simulink model "QCar2_DetailedScenario-2025a"  (R2025a)
settings: Solver=ode2  StartTime=0.0  StopTime=inf  FixedStep=1/100  RelTol=1e-3  EnableMultiTasking=on
model workspace (MAT data in the model file):
  XY_OFFSET : Simulink.Parameter (value not decoded)
  camera_rate : Simulink.Parameter (value not decoded)
  depth_rate : Simulink.Parameter (value not decoded)
  path_to_pickup : Simulink.Parameter (value not decoded)
  path_to_pickup_tight : Simulink.Parameter (value not decoded)
symbols that are objects in the model workspace (value not decoded): camera_rate, depth_rate, path_to_pickup, XY_OFFSET
undefined symbols (not defined in the file or in its folder): gcbh, HIL, JPEG, Point, qc_get_step_size, Video3D, video_display_show
libraries: quarc_library x37, simulink x16
(part 2 of 3)

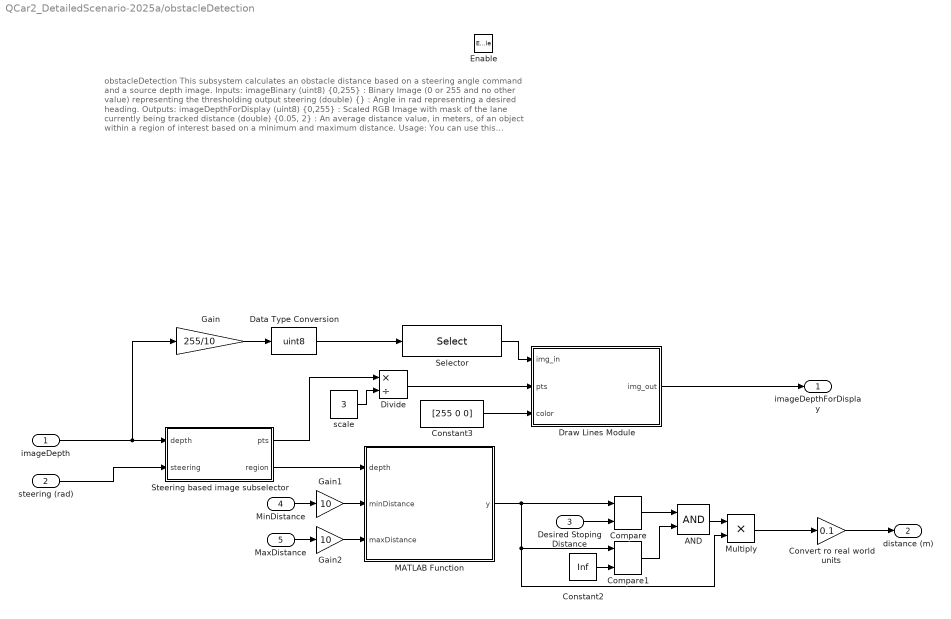
== system QCar2_DetailedScenario-2025a/obstacleDetection ==
  note: obstacleDetection
      | This subsystem calculates an obstacle distance based on a steering angle command and a source depth image.
      |
      | Inputs:
      | imageBinary (uint8) {0,255} : Binary Image (0 or 255 and no other value) representing the thresholding output
      | steering (double) {} : Angle in rad representing a desired heading.
      |
      | Outputs:
      | imageDepthForDisplay (uint8) {0,255} : Scaled RGB Image with mask of the lane currently being tracked
      | distance (double) {0.05, 2} : An average distance value, in meters, of an object within a region of interest based on a minimum and maximum distance.
      |
      | Usage:
      |
      | You can use this subsystem to determine if the desired heading angle will cause the car to colllide with an obstacle by examining the distances from a region of interest within the depth image and calculating how far the obstacle is.
  imageDepth : Inport
  steering (rad) : Inport  Port=2
  Desired Stoping Distance : Inport  Port=3
  MinDistance : Inport  Port=4
  MaxDistance : Inport  Port=5
  Enable : EnablePort  PropagateVarSize=During execution
  AND : Logic  AllPortsSameDT=off  OutDataTypeStr=boolean
  Compare : quarc_library/Logic Operations/Compare  operator=>=  output_data_type=boolean
      settings: SourceProductName=QUARC Targets
  Compare1 : quarc_library/Logic Operations/Compare  operator=<  output_data_type=boolean
      settings: SourceProductName=QUARC Targets
  Constant2 : Constant  Value=Inf
  Constant3 : Constant  Value=[255 0 0]
  Convert ro real world units : Gain  Gain=0.1
  Data Type Conversion : DataTypeConversion  OutDataTypeStr=uint8  SaturateOnIntegerOverflow=off  RndMeth=Floor
  Divide : Product  Inputs=*/  OutDataTypeStr=Inherit: Inherit via back propagation
  Draw Lines Module : MATLAB Function  TreatAsAtomicUnit=on
  Gain : Gain  Gain=255/10
  Gain1 : Gain  Gain=10
  Gain2 : Gain  Gain=10
  MATLAB Function : MATLAB Function  TreatAsAtomicUnit=on
  Multiply : Product
  Selector : Selector  NumberOfDimensions=2  InputPortWidth=3  IndexOptions=Index vector (dialog),Index vector (dialog)  Indices=[1:3:360],[1:3:640]  OutputSizes=1,1
  Steering based image subselector : MATLAB Function  TreatAsAtomicUnit=on
  scale : Constant  Value=3
  imageDepthForDisplay : Outport  VectorParamsAs1DForOutWhenUnconnected=off
  distance (m) : Outport  Port=2  VectorParamsAs1DForOutWhenUnconnected=off
  wires:
  Constant3/1 -> Draw Lines Module/3(color)
  Steering based image subselector/1(pts) -> Divide/1
  Steering based image subselector/2(region) -> MATLAB Function/1(depth)
  steering (rad)/1 -> Steering based image subselector/2(steering)
  Multiply/1 -> Convert ro real world units/1
  MaxDistance/1 -> Gain2/1
  MinDistance/1 -> Gain1/1
  MATLAB Function/1(y) -> Compare/1, Multiply/2, Compare1/1
  imageDepth/1 -> Steering based image subselector/1(depth), Gain/1
  Selector/1 -> Draw Lines Module/1(img_in)
  Data Type Conversion/1 -> Selector/1
  Divide/1 -> Draw Lines Module/2(pts)
  Draw Lines Module/1(img_out) -> imageDepthForDisplay/1
  scale/1 -> Divide/2
  Gain/1 -> Data Type Conversion/1
  Desired Stoping Distance/1 -> Compare/2
  Compare/1 -> AND/1
  Compare1/1 -> AND/2
  Constant2/1 -> Compare1/2
  AND/1 -> Multiply/1
  Convert ro real world units/1 -> distance (m)/1
  Gain1/1 -> MATLAB Function/2(minDistance)
  Gain2/1 -> MATLAB Function/3(maxDistance)

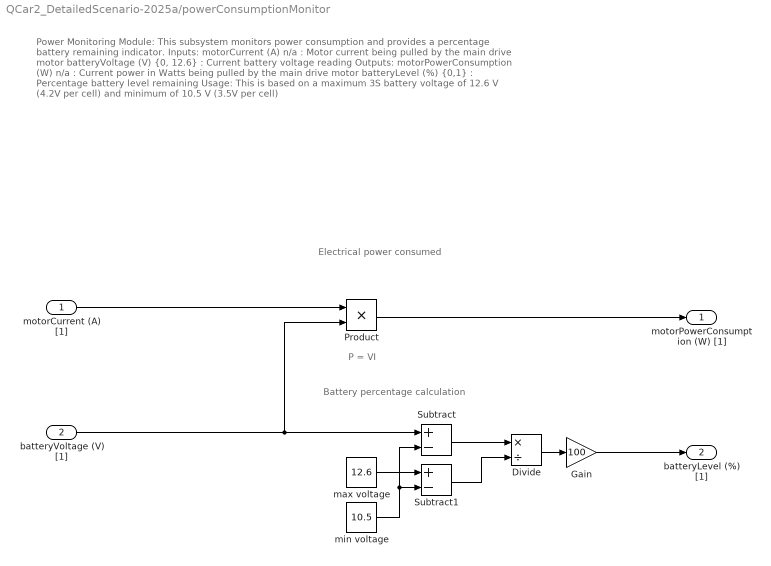
== system QCar2_DetailedScenario-2025a/powerConsumptionMonitor ==
  note: Battery percentage calculation
  note: P = VI
  note: Electrical
      | power
      | consumed
  note: Power Monitoring Module:
      |
      | This subsystem monitors power consumption and provides a percentage battery remaining indicator.
      |
      | Inputs:
      | motorCurrent (A) n/a : Motor current being pulled by the main drive motor
      | batteryVoltage (V) {0, 12.6} : Current battery voltage reading
      |
      | Outputs:
      | motorPowerConsumption (W) n/a : Current power in Watts being pulled by the main drive motor
      | batteryLevel (%) {0,1} : Percentage battery level remaining
      |
      | Usage:
      | This is based on a maximum 3S battery voltage of 12.6 V (4.2V per cell) and minimum of 10.5 V (3.5V per cell)
  motorCurrent (A) [1] : Inport
  batteryVoltage (V) [1] : Inport  Port=2
  Divide : Product  Inputs=*/
  Gain : Gain  Gain=100
  Product : Product
  Subtract : Sum  Inputs=+-
  Subtract1 : Sum  Inputs=+-
  max voltage : Constant  Value=12.6
  min voltage : Constant  Value=10.5
  motorPowerConsumption (W) [1] : Outport  VectorParamsAs1DForOutWhenUnconnected=off
  batteryLevel (%) [1] : Outport  Port=2  VectorParamsAs1DForOutWhenUnconnected=off
  wires:
  Divide/1 -> Gain/1
  Subtract1/1 -> Divide/2
  Gain/1 -> batteryLevel (%) [1]/1
  Product/1 -> motorPowerConsumption (W) [1]/1
  min voltage/1 -> Subtract/2, Subtract1/2
  motorCurrent (A) [1]/1 -> Product/1
  max voltage/1 -> Subtract1/1
  Subtract/1 -> Divide/1
  batteryVoltage (V) [1]/1 -> Subtract/1, Product/2

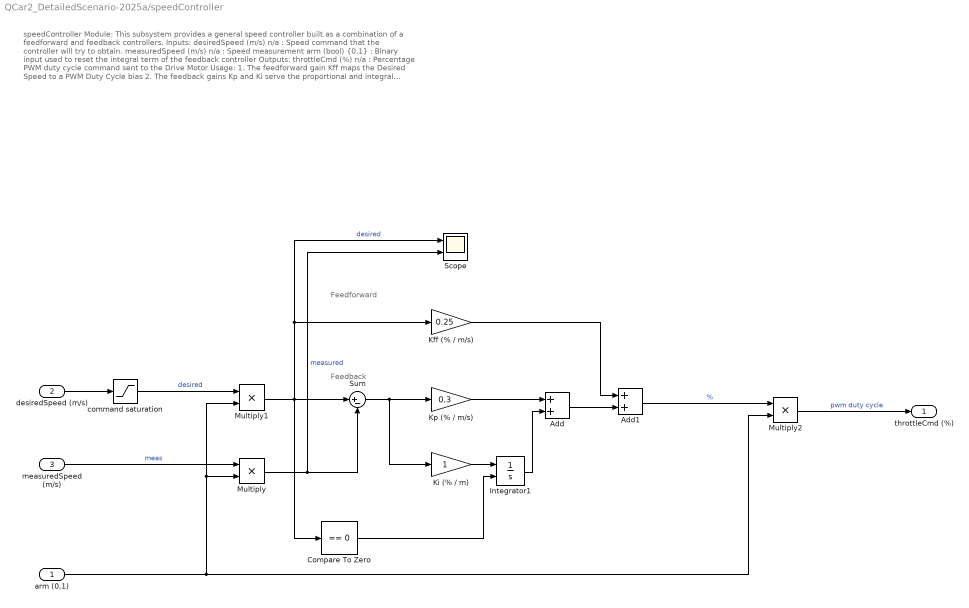
== system QCar2_DetailedScenario-2025a/speedController ==
  note: Feedforward
  note: Feedback
  note: speedController Module:
      |
      | This subsystem provides a general speed controller built as a combination of a feedforward and feedback controllers.
      |
      | Inputs:
      | desiredSpeed (m/s) n/a : Speed command that the controller will try to obtain.
      | measuredSpeed (m/s) n/a : Speed measurement
      | arm (bool) {0,1} : Binary input used to reset the integral term of the feedback controller
      |
      | Outputs:
      | throttleCmd (%) n/a : Percentage PWM duty cycle command sent to the Drive Motor
      |
      | Usage:
      | 1. The feedforward gain Kff maps the Desired Speed to a PWM Duty Cycle bias
      | 2. The feedback gains Kp and Ki serve the proportional and integral terms to output corrections to the PWM Duty Cycle so as to regulate the desired speed.
  arm (0,1) : Inport
  desiredSpeed (m/s) : Inport  Port=2
  measuredSpeed (m/s) : Inport  Port=3
  Add : Sum
  Add1 : Sum
  Compare To Zero : simulink/Logic and Bit Operations/Compare To Zero  relop===  OutDataTypeStr=boolean
  Integrator1 : Integrator  ExternalReset=either  LimitOutput=on  UpperSaturationLimit=0.4  LowerSaturationLimit=-0.4
  Kff (% / m/s) : Gain  Gain=0.25
  "Ki (% / m) " : Gain
  Kp (% / m/s) : Gain  Gain=0.3
  Multiply : Product
  Multiply1 : Product
  Multiply2 : Product
  Scope : Scope  NumInputPorts=2
      settings: Title=Control Performance  ActiveDisplayYMinimum=1.4224  ActiveDisplayYMaximum=2.10565  YLabel=m/s
  Sum : Sum  Inputs=|+-
  command saturation : Saturate  UpperLimit=5  LowerLimit=-5
  throttleCmd (%) : Outport  VectorParamsAs1DForOutWhenUnconnected=off
  wires:
  command saturation/1 -> Multiply1/1  "desired"
  arm (0,1)/1 -> Multiply1/2, Multiply/2, Multiply2/2
  measuredSpeed (m/s)/1 -> Multiply/1  "meas"
  Multiply/1 -> Sum/2, Scope/2  "measured"
  Add/1 -> Add1/2
  Add1/1 -> Multiply2/1  "%"
  Multiply1/1 -> Compare To Zero/1, Sum/1, Kff (% / m/s)/1, Scope/1  "desired"
  Integrator1/1 -> Add/2
  Multiply2/1 -> throttleCmd (%)/1  "pwm duty cycle"
  Kp (% / m/s)/1 -> Add/1
  Compare To Zero/1 -> Integrator1/2
  Kff (% / m/s)/1 -> Add1/1
  Sum/1 -> "Ki (% / m) "/1, Kp (% / m/s)/1
  "Ki (% / m) "/1 -> Integrator1/1
  desiredSpeed (m/s)/1 -> command saturation/1

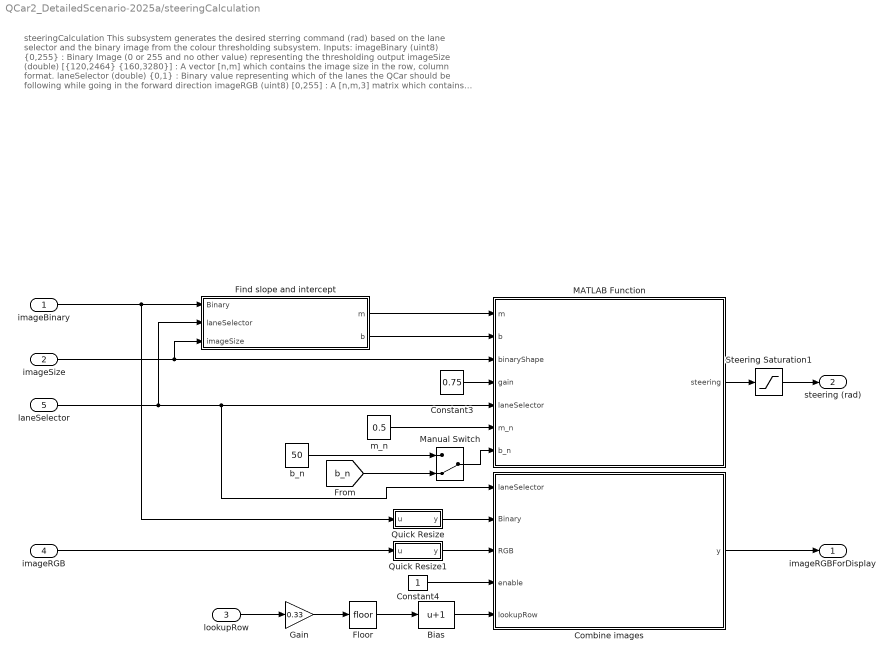
== system QCar2_DetailedScenario-2025a/steeringCalculation ==
  note: steeringCalculation
      | This subsystem generates the desired sterring command (rad) based on the lane selector and the binary image from the colour thresholding subsystem.
      |
      | Inputs:
      | imageBinary (uint8) {0,255} : Binary Image (0 or 255 and no other value) representing the thresholding output
      | imageSize (double) [{120,2464} {160,3280}] : A vector [n,m] which contains the image size in the row, column format.
      | laneSelector (double) {0,1} : Binary value representing which of the lanes the QCar should be following while going in the forward direction
      | imageRGB (uint8) [0,255] : A [n,m,3] matrix which contains RGB values of an image in uint8 format
      |
      | Outputs:
      | steering (double) {-0.5,0.5} : Angle in rad representing the desired steering command based on the linearPolyFit
      | imageRGBForDisplay (uint8) {0,255} : A [n,m,3] matrix representing an RGB Image with mask of the lane currently being tracked
      |
      | Usage:
      |
      | This module can be used to generate a desired steering angle based on a thresheld image. A linear polygonal fit is used to generate a slope based on the equation y = mx+b whose slope and y intercept will define the steering angle commanded up to 0.5 (rad). The RGB image is a combination of the binary image holding information of the lane being followed, and a scaled version of the original RGB image.
  imageBinary : Inport
  imageSize : Inport  Port=2
  lookupRow : Inport  Port=3
  imageRGB : Inport  Port=4
  laneSelector : Inport  Port=5
  Bias : Bias  Bias=1  SaturateOnIntegerOverflow=off
  Combine images : MATLAB Function  TreatAsAtomicUnit=on
  Constant3 : Constant  Value=0.75
  Constant4 : Constant
  Find slope and intercept : MATLAB Function  TreatAsAtomicUnit=on
  Floor : Rounding
  Gain : Gain  Gain=0.33
  MATLAB Function : MATLAB Function  TreatAsAtomicUnit=on
  Manual Switch : ManualSwitch  CurrentSetting=0
  Quick Resize : MATLAB Function  TreatAsAtomicUnit=on
  Quick Resize1 : MATLAB Function  TreatAsAtomicUnit=on
  Steering Saturation1 : Saturate
  b_n : Constant  Value=50
  m_n : Constant  Value=0.5
  imageRGBForDisplay : Outport  VectorParamsAs1DForOutWhenUnconnected=off
  steering (rad) : Outport  Port=2  VectorParamsAs1DForOutWhenUnconnected=off
  wires:
  Find slope and intercept/1(m) -> MATLAB Function/1(m)
  laneSelector/1 -> MATLAB Function/5(laneSelector), Combine images/1(laneSelector), Find slope and intercept/2(laneSelector)
  MATLAB Function/1(steering) -> Steering Saturation1/1
  Constant3/1 -> MATLAB Function/4(gain)
  imageBinary/1 -> Quick Resize/1(u), Find slope and intercept/1(Binary)
  Find slope and intercept/2(b) -> MATLAB Function/2(b)
  Constant4/1 -> Combine images/4(enable)
  Quick Resize/1(y) -> Combine images/2(Binary)
  Quick Resize1/1(y) -> Combine images/3(RGB)
  Combine images/1(y) -> imageRGBForDisplay/1
  imageRGB/1 -> Quick Resize1/1(u)
  Steering Saturation1/1 -> steering (rad)/1
  Gain/1 -> Floor/1
  imageSize/1 -> Find slope and intercept/3(imageSize), MATLAB Function/3(binaryShape)
  lookupRow/1 -> Gain/1
  Bias/1 -> Combine images/5(lookupRow)
  Floor/1 -> Bias/1
  b_n/1 -> Manual Switch/1
  Manual Switch/1 -> MATLAB Function/7(b_n)
  [b_n] -> Manual Switch/2
  m_n/1 -> MATLAB Function/6(m_n)

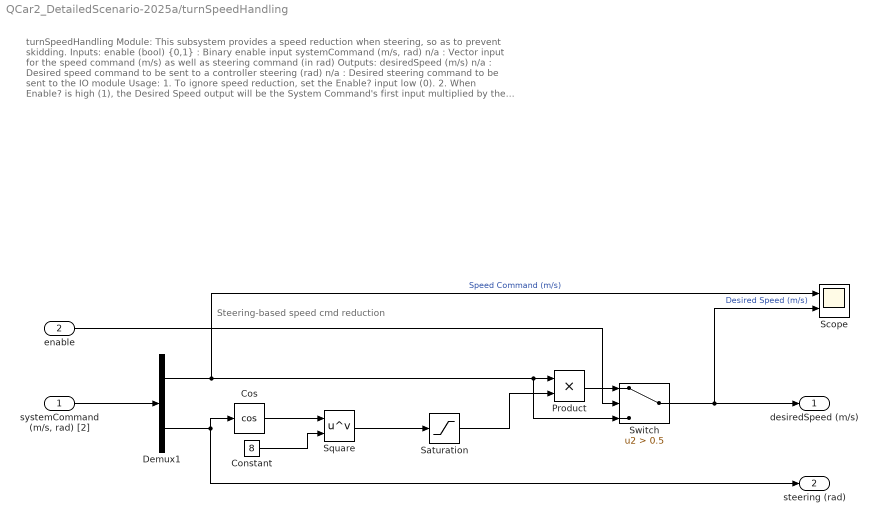
== system QCar2_DetailedScenario-2025a/turnSpeedHandling ==
  note: turnSpeedHandling Module:
      |
      | This subsystem provides a speed reduction when steering, so as to prevent skidding.
      |
      | Inputs:
      | enable (bool) {0,1} : Binary enable input
      | systemCommand (m/s, rad) n/a : Vector input for the speed command (m/s) as well as steering command (in rad)
      |
      | Outputs:
      | desiredSpeed (m/s) n/a : Desired speed command to be sent to a controller
      | steering (rad) n/a : Desired steering command to be sent to the IO module
      |
      | Usage:
      | 1. To ignore speed reduction, set the Enable? input low (0).
      | 2. When Enable? is high (1), the Desired Speed output will be the System Command's first input multiplied by the cosine of the steering. Note that the lower limit of this reduction is set to 50% of the speed command input.
  note: Steering-based speed cmd reduction
  "systemCommand (m/s, rad) [2]" : Inport
  enable : Inport  Port=2
  Constant : Constant  Value=8
  Cos : Trigonometry  Operator=cos
  Demux1 : Demux  Outputs=2
  Product : Product
  Saturation : Saturate  UpperLimit=1  LowerLimit=0.5
  Scope : Scope  NumInputPorts=2
      settings: Title=Turn-Speed Handling  ActiveDisplayYMinimum=-2  ActiveDisplayYMaximum=2  YLabel=m/s  DataLoggingVariableName=ScopeData2
  Square : Math  Operator=pow  SignedPower=on
  Switch : Switch  Criteria=u2 > Threshold  Threshold=0.5  SaturateOnIntegerOverflow=off  InputSameDT=off
  desiredSpeed (m/s) : Outport  VectorParamsAs1DForOutWhenUnconnected=off
  steering (rad) : Outport  Port=2  VectorParamsAs1DForOutWhenUnconnected=off
  wires:
  Cos/1 -> Square/1
  Switch/1 -> desiredSpeed (m/s)/1, Scope/2  "Desired Speed (m/s)"
  Product/1 -> Switch/1
  Saturation/1 -> Product/2
  Demux1/1 -> Product/1, Switch/3, Scope/1  "Speed Command (m/s)"
  "systemCommand (m/s, rad) [2]"/1 -> Demux1/1
  enable/1 -> Switch/2
  Constant/1 -> Square/2
  Demux1/2 -> steering (rad)/1, Cos/1
  Square/1 -> Saturation/1

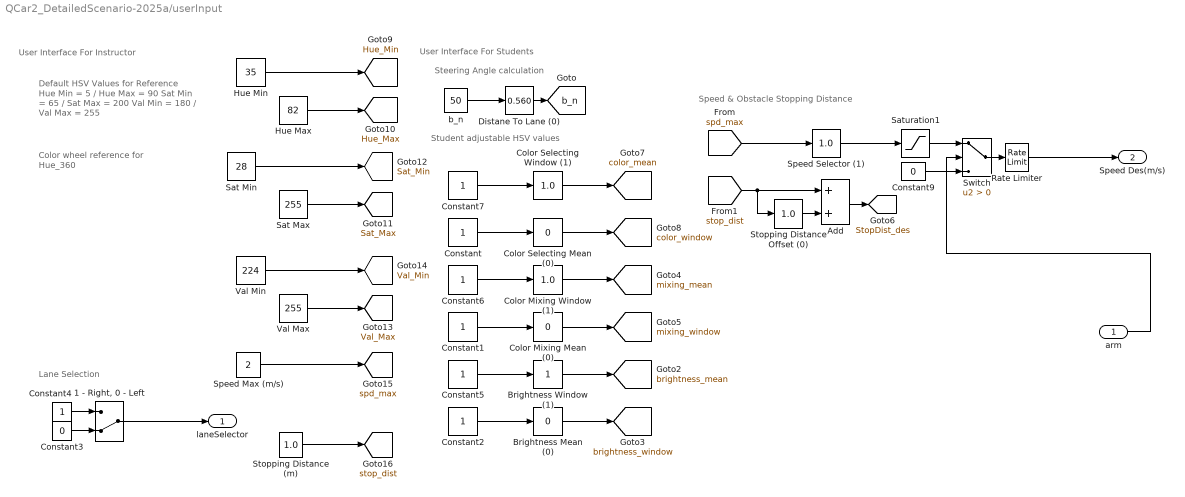
== system QCar2_DetailedScenario-2025a/userInput ==
  note: Default HSV Values for Reference
      | Hue Min = 5 / Hue Max = 90
      | Sat Min = 65 / Sat Max = 200
      | Val Min = 180 / Val Max = 255
  note: User Interface For Instructor
  note: Student adjustable HSV values
  note: Lane Selection
  note: Steering Angle calculation
  note: User Interface For Students
  note: Speed & Obstacle Stopping Distance
  note: Color wheel
      | reference
      | for Hue_360
  arm : Inport  OutDataTypeStr=boolean
  "1 - Right, 0 - Left" : ManualSwitch  CurrentSetting=0
  Add : Sum
  Brightness Mean (0) : simulink/Math Operations/Slider Gain  gain=0  low=-1  high=1
  Brightness Window (1) : simulink/Math Operations/Slider Gain  gain=1  low=0  high=1
  Color Mixing Mean (0) : simulink/Math Operations/Slider Gain  gain=0  low=-1  high=1
  Color Mixing Window (1) : simulink/Math Operations/Slider Gain  gain=1.0  low=0  high=1
  Color Selecting Mean (0) : simulink/Math Operations/Slider Gain  gain=0  low=-1  high=1
  Color Selecting Window (1) : simulink/Math Operations/Slider Gain  gain=1.0  low=0  high=1
  Constant{,1..2,4..7} (7 alike) : Constant
  Constant3 : Constant  Value=0
  Constant9 : Constant  Value=0
  "Distane To Lane (0) " : simulink/Math Operations/Slider Gain  gain=0.560  low=0  high=1
  Hue Max : Constant  Value=82
  Hue Min : Constant  Value=35
  Rate Limiter : RateLimiter  FallingSlewLimit=-Inf  SampleTimeMode=inherited
  Sat Max : Constant  Value=255
  Sat Min : Constant  Value=28
  Saturation1 : Saturate  UpperLimit=1  LowerLimit=0
  Speed Max (m/s) : Constant  Value=2
  Speed Selector (1) : simulink/Math Operations/Slider Gain  gain=1.0  low=0  high=1
  Stopping Distance (m) : Constant  Value=1.0
  Stopping Distance Offset (0) : simulink/Math Operations/Slider Gain  gain=1.0  low=0  high=1
  Switch : Switch  Criteria=u2 > Threshold  SaturateOnIntegerOverflow=off  InputSameDT=off
  Val Max : Constant  Value=255
  Val Min : Constant  Value=224
  b_n : Constant  Value=50
  laneSelector : Outport  VectorParamsAs1DForOutWhenUnconnected=off
  Speed Des(m/s) : Outport  Port=2  VectorParamsAs1DForOutWhenUnconnected=off
  tag scope: Hue_Max=global, Hue_Min=global, Sat_Max=global, Sat_Min=global, StopDist_des=global, Val_Max=global, Val_Min=global, b_n=global, brightness_mean=global, brightness_window=global, color_mean=global, color_window=global, mixing_mean=global, mixing_window=global, spd_max=global, stop_dist=global
  wires:
  Constant3/1 -> "1 - Right, 0 - Left"/2
  b_n/1 -> "Distane To Lane (0) "/1
  Constant4/1 -> "1 - Right, 0 - Left"/1
  Switch/1 -> Rate Limiter/1
  Constant9/1 -> Switch/3
  [spd_max] -> Speed Selector (1)/1
  Saturation1/1 -> Switch/1
  "1 - Right, 0 - Left"/1 -> laneSelector/1
  Rate Limiter/1 -> Speed Des(m/s)/1
  "Distane To Lane (0) "/1 -> [b_n]
  Color Mixing Window (1)/1 -> [mixing_mean]
  Constant/1 -> Color Selecting Mean (0)/1
  Constant2/1 -> Brightness Mean (0)/1
  Constant5/1 -> Brightness Window (1)/1
  Constant1/1 -> Color Mixing Mean (0)/1
  Color Selecting Mean (0)/1 -> [color_window]
  Brightness Window (1)/1 -> [brightness_mean]
  Color Selecting Window (1)/1 -> [color_mean]
  Brightness Mean (0)/1 -> [brightness_window]
  Color Mixing Mean (0)/1 -> [mixing_window]
  Constant6/1 -> Color Mixing Window (1)/1
  Constant7/1 -> Color Selecting Window (1)/1
  Hue Min/1 -> [Hue_Min]
  Sat Min/1 -> [Sat_Min]
  Val Min/1 -> [Val_Min]
  Hue Max/1 -> [Hue_Max]
  Sat Max/1 -> [Sat_Max]
  Val Max/1 -> [Val_Max]
  Speed Selector (1)/1 -> Saturation1/1
  Speed Max (m/s)/1 -> [spd_max]
  Stopping Distance (m)/1 -> [stop_dist]
  [stop_dist] -> Stopping Distance Offset (0)/1, Add/1
  Stopping Distance Offset (0)/1 -> Add/2
  Add/1 -> [StopDist_des]
  arm/1 -> Switch/2

== system QCar2_DetailedScenario-2025a/basicQCarIO/Video Compressed Display ==
  In1 : Inport
  Channel : quarc_library/Signal Routing/Channel  channel=3  buffer_size=1
  Image Compress : quarc_library/Image Processing/Generic/Image Compress  algorithm=JPEG  source=Internal dialog parameter  quality=quality  output_dim=-1
  Video Display : quarc_library/Multimedia/Video Display  Tag=QCar2_DetailedScenario/basicQCarIO/Video Compressed Display/Video Display  sample_time=sample_time  use_hardware=on
  wires:
  Image Compress/1 -> Channel/1
  In1/1 -> Image Compress/1
  Channel/1 -> Video Display/1

== system QCar2_DetailedScenario-2025a/basicQCarIO/captureLIDAR ==
  note: captureLIDAR Module:
      |
      | This subsystem reads the LIDAR data from the QCar. This module reads 720 points per revolution at 30 Hz (30 scans per s).
      |
      | Outputs:
      | distances (m) n/a : Distances to obstacles measured
      | headings (rad) n/a : Headings at which distances were measured
  note: LIDAR Capture, and heading adjustment
  "Change +x to front of QCar " : Bias  SaturateOnIntegerOverflow=off
  Change to CCW rotation : Gain  Gain=-1
  Ranging Sensor : quarc_library/Devices/Third-Party/Sensors/Ranging Sensor  sensor_type=RPLidar LIDAR  uri=tcpip://localhost:18966  ranging_distance=Long  timing_budget=0.033  measurement_period=0.0001  output_mode=Fixed-size output  samples_per_revolution=360  max_distance=Inf  max_angle=5  sample_time=qc_get_step_size  show_versions=off  active=on
      settings: SourceProductName=QUARC Targets
  Terminator{,1..3} (4 alike) : Terminator
  distances (m) : Outport  VectorParamsAs1DForOutWhenUnconnected=off
  headings (rad) : Outport  Port=2  VectorParamsAs1DForOutWhenUnconnected=off
  wires:
  Ranging Sensor/1 -> distances (m)/1
  "Change +x to front of QCar "/1 -> headings (rad)/1
  Ranging Sensor/3 -> Change to CCW rotation/1
  Ranging Sensor/2 -> Terminator/1
  Change to CCW rotation/1 -> "Change +x to front of QCar "/1
  Ranging Sensor/5 -> Terminator3/1
  Ranging Sensor/6 -> Terminator1/1
  Ranging Sensor/4 -> Terminator2/1

== system QCar2_DetailedScenario-2025a/basicQCarIO/monitorTiming  ==
  note: Timing Performance
  note: monitorTiming Module:
      |
      | This subsystem provides three timing signals for any given rate in your model.
      |
      | Outputs:
      | timing (s) n/a : Sample time, sample time reference and computation time in seconds.
      |
      | Usage:
      | Set the 'Sample time (seconds)' parameter in all three blocks below to the same number. This will provide the actual sample time at each time step, the reference sample time that is being targeted as well as the computation time of that particular loop in the model into one vector signal for scoping.
  Computation Time : quarc_library/Sources/Time/Computation Time  sample_time=qc_get_step_size  use_model=on  use_cpu_time=off
  Constant : Constant  Value=qc_get_step_size
  Mux : Mux  Inputs=3
  Sample Time : quarc_library/Sources/Time/Sample Time  Priority=-99  sample_time=qc_get_step_size
  timing (s) : Outport  VectorParamsAs1DForOutWhenUnconnected=off
  wires:
  Mux/1 -> timing (s)/1
  Computation Time/1 -> Mux/3  "computation time"
  Sample Time/1 -> Mux/1  "actual sample time"
  Constant/1 -> Mux/2  "reference"

== system QCar2_DetailedScenario-2025a/basicQCarIO/odometry ==
  v_in : Inport
  steer_in : Inport  Port=2
  Ts_const : Constant  Value=0.02
  odometry_step : MATLAB Function  TreatAsAtomicUnit=on
  state_delay : UnitDelay  InitialCondition=[0;0;0]  SampleTime=-1  HasFrameUpgradeWarning=on
  pose_out : Outport
  wires:
  state_delay/1 -> odometry_step/1(prev_state)
  v_in/1 -> odometry_step/2(v)
  steer_in/1 -> odometry_step/3(steer)
  Ts_const/1 -> odometry_step/4(Ts)
  odometry_step/1(pose_next) -> state_delay/1, pose_out/1

== system QCar2_DetailedScenario-2025a/basicQCarIO/pointCloud ==
  note: Convert LIDAR information to Point Cloud Image
  note: pointCloud Module:
      |
      | This subsystem generates a point cloud image based on LIDAR data.
      |
      | Inputs:
      | distances (m) n/a : Distances measured by LIDAR
      | headings (rad) n/a : Headings at which distances are measured
      |
      | Outputs:
      | map (px) {0, 1} : 400 x 400 point cloud image
      |
      | Usage:
      | The data is dynamically saturated based on the maximumDistance (m) constant. To prevent a circle with radius being the maximumDistance showing up in the point cloud as a result of this saturation, data points corresponding to this are dropped in the findXYContour function. The function contourToPointCloud updates pixels in the map to 1 at new locations, and decays older data at the rate specified by the decay parameter.
  distances (m) : Inport
  heading (rad) : Inport  Port=2
  Constant1 : Constant  Value=0
  Saturation Dynamic : simulink/Discontinuities/Saturation Dynamic  OutMin=[]  OutMax=[]  OutDataTypeStr=Inherit: Same as second input  OutDataType=fixdt(1, 16)  OutScaling=2^-10  DoSatur=off
  contourToPointCloud : MATLAB Function  TreatAsAtomicUnit=on
  decay : Constant  Value=0
  findXYContour : MATLAB Function  TreatAsAtomicUnit=on
  maximumDistance (m) : Constant  Value=4
  map : Outport  VectorParamsAs1DForOutWhenUnconnected=off
  wires:
  distances (m)/1 -> Saturation Dynamic/2
  contourToPointCloud/1(mapOut) -> map/1
  Saturation Dynamic/1 -> findXYContour/1(distances)
  maximumDistance (m)/1 -> findXYContour/3(d_max), Saturation Dynamic/1
  Constant1/1 -> Saturation Dynamic/3
  decay/1 -> contourToPointCloud/3(decay)
  findXYContour/1(X) -> contourToPointCloud/1(X)
  findXYContour/2(Y) -> contourToPointCloud/2(Y)
  heading (rad)/1 -> findXYContour/2(heading)

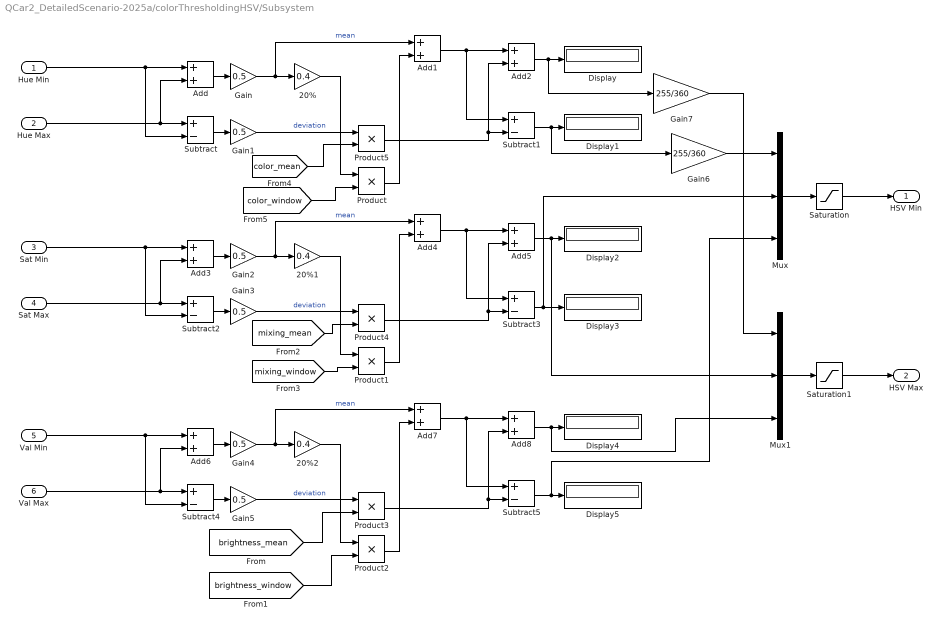
== system QCar2_DetailedScenario-2025a/colorThresholdingHSV/Subsystem ==
  Hue Min : Inport
  Hue Max : Inport  Port=2
  Sat Min : Inport  Port=3
  Sat Max : Inport  Port=4
  Val Min : Inport  Port=5
  Val Max : Inport  Port=6
  20% : Gain  Gain=0.4
  20%1 : Gain  Gain=0.4
  20%2 : Gain  Gain=0.4
  Add{,1..8} (9 alike) : Sum
  Display{,1..5} (6 alike) : Display
  Gain{,1..5} (6 alike) : Gain  Gain=0.5
  Gain6 : Gain  Gain=255/360
  Gain7 : Gain  Gain=255/360
  Mux : Mux  Inputs=3
  Mux1 : Mux  Inputs=3
  Product{,1..5} (6 alike) : Product
  Saturation : Saturate  UpperLimit=[255 255 255]  LowerLimit=[0 0 0]
  Saturation1 : Saturate  UpperLimit=[255 255 255]  LowerLimit=[0 0 0]
  Subtract{,1..5} (6 alike) : Sum  Inputs=+-
  HSV Min : Outport  VectorParamsAs1DForOutWhenUnconnected=off
  HSV Max : Outport  Port=2  VectorParamsAs1DForOutWhenUnconnected=off
  wires:
  Product1/1 -> Add4/2
  Val Min/1 -> Add6/1, Subtract4/2
  Mux/1 -> Saturation/1
  Subtract1/1 -> Gain6/1, Display1/1
  Subtract4/1 -> Gain5/1
  Add1/1 -> Subtract1/1, Add2/1
  Product3/1 -> Add8/2, Subtract5/2
  Product2/1 -> Add7/2
  Gain4/1 -> 20%2/1, Add7/1  "mean"
  Add2/1 -> Gain7/1, Display/1
  Subtract3/1 -> Mux/2, Display3/1
  Subtract5/1 -> Mux/3, Display5/1
  Gain/1 -> 20%/1, Add1/1  "mean"
  Sat Min/1 -> Subtract2/2, Add3/1
  Subtract2/1 -> Gain3/1
  Product5/1 -> Add2/2, Subtract1/2
  Gain5/1 -> Product3/1  "deviation"
  Add5/1 -> Mux1/2, Display2/1
  Gain2/1 -> Add4/1, 20%1/1  "mean"
  Add8/1 -> Mux1/3, Display4/1
  Product/1 -> Add1/2
  Subtract/1 -> Gain1/1
  Product4/1 -> Subtract3/2, Add5/2
  Add4/1 -> Add5/1, Subtract3/1
  Add7/1 -> Subtract5/1, Add8/1
  Sat Max/1 -> Subtract2/1, Add3/2
  20%1/1 -> Product1/1
  [brightness_mean] -> Product3/2
  Mux1/1 -> Saturation1/1
  Add3/1 -> Gain2/1
  [mixing_mean] -> Product4/2
  Hue Min/1 -> Add/1, Subtract/2
  Hue Max/1 -> Add/2, Subtract/1
  Gain3/1 -> Product4/1  "deviation"
  Val Max/1 -> Add6/2, Subtract4/1
  20%2/1 -> Product2/1
  Add6/1 -> Gain4/1
  [color_window] -> Product/2
  [color_mean] -> Product5/2
  20%/1 -> Product/1
  Add/1 -> Gain/1
  Gain1/1 -> Product5/1  "deviation"
  [mixing_window] -> Product1/2
  [brightness_window] -> Product2/2
  Saturation/1 -> HSV Min/1
  Saturation1/1 -> HSV Max/1
  Gain6/1 -> Mux/1
  Gain7/1 -> Mux1/1

== matlab function QCar2_DetailedScenario-2025a/steeringCalculation/MATLAB Function ==
  data: m input; steering output; b input; binaryShape input; gain input; laneSelector input; m_n input; b_n input
function steering = fcn(m, b, binaryShape, gain, laneSelector, m_n, b_n)
 
% y = mx + b

current_x = (binaryShape(1) - b)/m;
nominal_x = (binaryShape(1) - b_n)/m_n;
if laneSelector
    steering = -gain*(nominal_x - current_x)/binaryShape(2);
else
    steering = gain*(nominal_x - current_x)/binaryShape(2);
end

== matlab function QCar2_DetailedScenario-2025a/steeringCalculation/Quick Resize ==
  data: u input; y output
function y = quickResize(u)

scale = 3;
    if length(size(u)) == 3
        y = u(1:scale:end, 1:scale:end, :);
    else
        y = u(1:scale:end, 1:scale:end);
    end

end

== matlab function QCar2_DetailedScenario-2025a/steeringCalculation/Combine images ==
  data: laneSelector input; Binary input; RGB input; y output size=[137,274,3]; enable input; lookupRow input
function y = laneMask(laneSelector, Binary, RGB, enable, lookupRow)

y = RGB;
[ROW, COL, ~] = size(y);
[binRow, ~] = size(Binary);
binarySection = Binary(binRow-(length(lookupRow:ROW))+1:binRow,:);
if enable
    if laneSelector
        section = RGB(lookupRow:ROW, COL*(2/3) + 1:COL, :);
        y(lookupRow:ROW, int16(COL*(2/3)) + 1:COL, 1) = ((255 - binarySection)/255).*section(:,:,1) + (binarySection).*section(:, :, 1);
        y(lookupRow:ROW, int16(COL*(2/3)) + 1:COL, 2) = ((255 - binarySection)/255).*section(:,:,2);
        y(lookupRow:ROW, int16(COL*(2/3)) + 1:COL, 3) = ((255 - binarySection)/255).*section(:,:,3);
    else
        section = RGB(lookupRow:ROW, 1:COL/3, :);
        y(lookupRow:ROW, 1:int16(COL/3), 1) = ((255 - binarySection)/255).*section(:,:,1) + (binarySection).*section(:, :, 1);
        y(lookupRow:ROW, 1:int16(COL/3), 2) = ((255 - binarySection)/255).*section(:,:,2);
        y(lookupRow:ROW, 1:int16(COL/3), 3) = ((255 - binarySection)/255).*section(:,:,3);
    end
end

== matlab function QCar2_DetailedScenario-2025a/obstacleDetection/MATLAB Function ==
  data: depth input; y output; minDistance input; maxDistance input
function y = calculateDistance(depth, minDistance, maxDistance)

% This function drops depth data when outside the minDistance:maxDistance
% bounds and then averages the result. 

% u_flat = reshape(depth, 1, []);
% u_flat(u_flat < minDistance) = [];
% u_flat(u_flat > maxDistance) = [];
% y = mean(mean(u_flat));


u_flat = depth(depth <maxDistance);

u_flat  = depth(u_flat>minDistance);

y = mean(u_flat);

== matlab function QCar2_DetailedScenario-2025a/obstacleDetection/Steering based image subselector ==
  data: pts output; depth input; region output; steering input
function [pts, region] = drawBox(depth, steering)
% Input: 640 x 360
mark = round(320 - (steering*260/0.5));
starting_index = mark+1-60;
region = double(depth(121:240, starting_index : starting_index + 119));
pts = [ 101, mark+1-60; 101, mark+60; 220, mark+60; 220, mark+1-60; 101, mark+1-60];

== matlab function QCar2_DetailedScenario-2025a/steeringCalculation/Quick Resize1 ==
  data: u input; y output
function y = quickResize(u)

scale = 3;
    if length(size(u)) == 3
        y = u(1:scale:end, 1:scale:end, :);
    else
        y = u(1:scale:end, 1:scale:end);
    end

end

== matlab function QCar2_DetailedScenario-2025a/automatedDriving/MATLAB Function ==
  data: obstacle_distance input; speed_cmd output; stop_distance input; nominal_tracking_distance input; nominal_speed input
function speed_cmd = adaptive_cruise_control(obstacle_distance, stop_distance, nominal_tracking_distance, nominal_speed)

speed_cmd = nominal_speed;

if obstacle_distance < stop_distance
    speed_cmd = 0;
    
elseif obstacle_distance < nominal_tracking_distance
    speed_cmd = nominal_speed/(nominal_tracking_distance-stop_distance)*obstacle_distance...
              - nominal_speed/(nominal_tracking_distance-stop_distance)*stop_distance;

end

== matlab function QCar2_DetailedScenario-2025a/MATLAB Function ==
  data: imageRGB input; imageToThreshold output; laneSelector input; lookupRow input; imageSize output
function [imageToThreshold, imageSize]  = imageSelector(imageRGB, laneSelector, lookupRow)

[ROW, COL, ~] = size(imageRGB);
% imageToThreshold = uint8(zeros(ROW/2+1,COL/3,3));
if laneSelector
    imageToThreshold = imageRGB(round(ROW/2)+1:ROW, round(COL*(2/3)) + 1:COL, :);
else
    imageToThreshold = imageRGB(round(ROW/2)+1:ROW, 1:round(COL/3), :);
end
imageToThreshold(1: round(ROW/2) - (ROW - lookupRow + 1),:,:) = 0;
imageSize = [ROW - lookupRow + 1, round(COL/3)];

== matlab function QCar2_DetailedScenario-2025a/maskArea ==
  data: u input; area output
function area = maskArea(u)
% u is logical or uint8 binary image
area = sum(u(:) ~= 0);
end

== matlab function QCar2_DetailedScenario-2025a/basicQCarIO/odometry/odometry_step ==
  data: prev_state input; pose_next output; v input; steer input; Ts input
function pose_next = odometry_step(prev_state, v, steer, Ts)
% prev_state: [x; y; yaw]
% v: longitudinal velocity (m/s)
% steer: front wheel steering angle (rad)
% Ts: sample time (s)
% Returns pose_next: [x; y; yaw]

% Parameters
L = 0.26; % wheelbase (m) - tune for your QCar

x = prev_state(1);
y = prev_state(2);
yaw = prev_state(3);

% Kinematic bicycle model
x_dot = v * cos(yaw);
y_dot = v * sin(yaw);
yaw_dot = (v / L) * tan(steer);

% Euler integration
x_next = x + Ts * x_dot;
y_next = y + Ts * y_dot;
yaw_next = yaw + Ts * yaw_dot;

% wrap yaw
yaw_next = atan2(sin(yaw_next), cos(yaw_next));

pose_next = [x_next; y_next; yaw_next];
end

== matlab function QCar2_DetailedScenario-2025a/waypointFollower ==
  settings: updateMethod=DISCRETE
  data: pose input; v_out output; path input; wp_idx_in input; omega_out output; reached output double size=1; wp_idx_out output
function [v_out, omega_out, reached, wp_idx_out] = waypointFollower(pose, path, wp_idx_in)
%#codegen
% Robust Pure Pursuit for QLabs/QCar with safe indexing and recovery.

% ===== Tunables =====
poseScaleXY = 10;     % 10 if pose is 1/10 QLabs, else 1

% Speed limits (QCar-safe)
v_max = 1.4;
v_min = 0.35;

% Steering/yaw-rate limits
omega_max = 0.90;

% Lookahead scheduling
Ld_min = 1.0;
Ld_max = 4.0;
kLd_v  = 1.4;         % Ld = Ld_min + kLd_v*v

% Curve speed limit
a_lat_max = 0.9;      % m/s^2

% Arrival
reach_dist = 8.0;     % 10x world? if your coords are 10x, keep 8.0; else 0.8

% Index search window / progress control
idx_window = 30;
maxStepFwd = 6;       % max forward index change per tick
maxStepBack = 2;      % allow small backward correction (fixes "stuck" / wrong idx)

% Off-path recovery
e_lat_slow   = 6.0;   % slow when farther than this
e_lat_freeze = 12.0;  % freeze progress when farther than this

% Smoothing / rate limit
tau_omega = 0.18;     % seconds
omega_rate_max = 2.0; % rad/s^2 (limit per second)
% =====================

% Defaults
v_out = 0.0;
omega_out = 0.0;
reached = 0.0;
wp_idx_out = double(wp_idx_in);

% Validate
if isempty(path) || size(path,2) ~= 2 || size(path,1) < 2
    return;
end

pose = double(pose(:));
if numel(pose) < 3
    return;
end
path = double(path);

% Pose
x = pose(1) * poseScaleXY;
y = pose(2) * poseScaleXY;
yaw = pose(3);

N = size(path,1);

% --- persistent waypoint index state (survives between calls) ---
persistent idx_state idx_init
if isempty(idx_init)
    idx_init = true;
    idx_state = 1;
end

% If caller provides a valid index, sync to it (optional)
idx_in = double(wp_idx_in);
if isfinite(idx_in) && (idx_in >= 1) && (idx_in <= N-1)
    % Only accept caller index if it isn't wildly behind (prevents reset-to-1 bugs)
    if idx_in > idx_state - 5
        idx_state = round(idx_in);
    end
end

idx0 = min(max(1, idx_state), N-1);

% Robust idx0
idx_in = double(wp_idx_in);
if ~isfinite(idx_in)
    idx_in = 1;
end
idx0 = min(max(1, round(idx_in)), N-1);

% dt (assume fixed-step sim ~0.02 if not provided)
dt = 0.02;

% persistent filter state
persistent omega_filt initialized
if isempty(initialized)
    initialized = true;
    omega_filt = 0.0;
end

% ---------- Reached check ----------
dx_end = path(N,1) - x;
dy_end = path(N,2) - y;
if hypot(dx_end, dy_end) <= reach_dist
    reached = 1.0;
    v_out = 0.0;
    omega_out = 0.0;
    wp_idx_out = double(N-1);
    return;
end

% ---------- 1) Find closest point on polyline near idx0 ----------
i_start = max(1, idx0 - idx_window);
i_end   = min(N-1, idx0 + idx_window);

best_d2 = 1e18;
best_i  = idx0;
best_t  = 0.0;
best_px = path(idx0,1);
best_py = path(idx0,2);

for i = i_start:i_end
    ax = path(i,1);   ay = path(i,2);
    bx = path(i+1,1); by = path(i+1,2);

    vx = bx-ax; vy = by-ay;
    wx = x-ax;  wy = y-ay;
    vv = vx*vx + vy*vy;

    if vv < 1e-9
        t = 0.0;
    else
        t = (wx*vx + wy*vy) / vv;
        if t < 0.0, t = 0.0; elseif t > 1.0, t = 1.0; end
    end

    px = ax + t*vx;
    py = ay + t*vy;

    dxp = x - px; dyp = y - py;
    d2 = dxp*dxp + dyp*dyp;

    if d2 < best_d2
        best_d2 = d2;
        best_i  = i;
        best_t  = t;
        best_px = px;
        best_py = py;
    end
end

e_lat = sqrt(best_d2);

% ---------- 2) FIXED: Stable, correct wp_idx_out ----------
% Use continuous progress along polyline (segment index + fraction)
s_prog = double(best_i) + double(best_t);     % in [1, N)
idx_des = floor(s_prog);                      % desired segment index

% If we're very near the end of the segment, advance the index
if best_t > 0.90
    idx_des = idx_des + 1;
end

% Clamp desired
idx_des = min(max(idx_des, 1), N-1);

% Freeze progress if far off path (your original behavior)
if e_lat > e_lat_freeze
    idx_des = idx0;
end

% Limit how fast index can move (forward AND backward)
delta = idx_des - idx0;
if delta >  maxStepFwd,  delta =  maxStepFwd;  end
if delta < -maxStepBack, delta = -maxStepBack; end

new_i = idx0 + delta;
new_i = min(max(new_i, 1), N-1);

% Recompute projection on chosen segment (critical)
ax = path(new_i,1);   ay = path(new_i,2);
bx = path(new_i+1,1); by = path(new_i+1,2);
vx = bx-ax; vy = by-ay;
wx = x-ax;  wy = y-ay;
vv = vx*vx + vy*vy;
if vv < 1e-9
    best_t = 0.0;
else
    best_t = (wx*vx + wy*vy)/vv;
    if best_t < 0.0, best_t = 0.0; elseif best_t > 1.0, best_t = 1.0; end
end
best_px = ax + best_t*vx;
best_py = ay + best_t*vy;

%wp_idx_out = double(new_i);

idx_state = new_i;           % store progress internally
wp_idx_out = double(new_i);  % output for logging / external use


% ---------- 3) Choose speed (preliminary) ----------
v_des = v_max;
if e_lat > e_lat_slow
    v_des = min(v_des, 0.7);
end
v_des = max(v_min, v_des);

% ---------- 4) Lookahead distance (speed-based) ----------
Ld = Ld_min + kLd_v * v_des;
Ld = min(max(Ld, Ld_min), Ld_max);

% ---------- 5) March along path by distance to get lookahead point ----------
remain = Ld;

sx = best_px; sy = best_py;
i = new_i;

bx = path(i+1,1); by = path(i+1,2);
seg_len = hypot(bx - sx, by - sy);

lx = bx; ly = by;

if seg_len >= remain
    u = remain / max(seg_len,1e-9);
    lx = sx + u*(bx - sx);
    ly = sy + u*(by - sy);
else
    remain = remain - seg_len;
    i = i + 1;
    while (remain > 0.0) && (i < N)
        ax = path(i,1);   ay = path(i,2);
        bx = path(i+1,1); by = path(i+1,2);
        seg_len = hypot(bx-ax, by-ay);

        if seg_len >= remain
            u = remain / max(seg_len,1e-9);
            lx = ax + u*(bx-ax);
            ly = ay + u*(by-ay);
            break;
        else
            remain = remain - seg_len;
            lx = bx; ly = by;
            i = i + 1;
        end
    end
    if i >= N
        lx = path(N,1);
        ly = path(N,2);
    end
end

% ---------- 6) Pure Pursuit control ----------
dx = lx - x;
dy = ly - y;

c = cos(yaw); s = sin(yaw);
x_r =  c*dx + s*dy;      % forward
y_r = -s*dx + c*dy;      % left

if x_r < 0.5
    omega_cmd = omega_max * sign(y_r);
    v_cmd = 0.5;
else
    kappa = 2.0 * y_r / max(Ld*Ld, 1e-6);

    v_curve = sqrt(a_lat_max / max(abs(kappa), 1e-6));
    v_cmd = min(v_des, v_curve);

    omega_cmd = kappa * v_cmd;
end

omega_cmd = max(-omega_max, min(omega_max, omega_cmd));

% ---------- 7) Rate limit + lowpass omega ----------
dOmega = omega_cmd - omega_filt;
maxStepOmega = omega_rate_max * dt;
if dOmega >  maxStepOmega, omega_cmd = omega_filt + maxStepOmega; end
if dOmega < -maxStepOmega, omega_cmd = omega_filt - maxStepOmega; end

aW = dt / max(tau_omega + dt, 1e-6);
omega_filt = (1-aW)*omega_filt + aW*omega_cmd;
omega = omega_filt;

% ---------- 8) Final speed schedule ----------
turnSlow = 1.0 - 0.6*min(abs(omega)/omega_max, 1.0);
v_cmd = v_cmd * turnSlow;

v_cmd = max(v_min, min(v_max, v_cmd));

if e_lat > e_lat_freeze
    v_cmd = min(v_cmd, 0.45);
end

v_out = double(v_cmd);
omega_out = double(omega);
reached = 0.0;
end

== matlab function QCar2_DetailedScenario-2025a/translatePath ==
  data: path_in input; path_out output; offset input
function path_out = translatePath(path_in, offset)
%#codegen
p = double(path_in);

% force offset into 1x2
o = double(offset(:)).';   % makes [2x1] -> [1x2], keeps [1x2] as [1x2]

% safety: if someone passed scalar, make it 1x2
if numel(o) == 1
    o = [o o];
end

% apply translation to every row
path_out = p + ones(size(p,1),1)*o;
end

== matlab function QCar2_DetailedScenario-2025a/basicQCarIO/pointCloud/contourToPointCloud ==
  data: X input size=720 [0..720]; mapOut output; Y input size=720; decay input
function mapOut = contourToPointCloud(X, Y, decay)
% Accumulate a 2D occupancy-like image from XY points (meters)
% X,Y can be vectors.

%#codegen

dim  = 400;   % image size dim x dim
gain = 50;    % pixels per meter

persistent mapInternal
if isempty(mapInternal)
    mapInternal = zeros(dim, dim);
else
    mapInternal = decay * mapInternal;
end

% Force column vectors
X = X(:);
Y = Y(:);

% 1-based center pixel
c = floor(dim/2) + 1;

% Map meters -> image coordinates
% col increases with +X, row decreases with +Y (typical image convention)
col = round(c + X * gain);
row = round(c - Y * gain);

% Keep only indices inside the image
valid = (row >= 1) & (row <= dim) & (col >= 1) & (col <= dim) ...
        & isfinite(row) & isfinite(col);

row = row(valid);
col = col(valid);

% If nothing valid, just output decayed map
if isempty(row)
    mapOut = mapInternal;
    return;
end

% Linear indexing (MATLAB is column-major): idx = row + (col-1)*dim
idx = row + (col - 1) * dim;

mapInternal(idx) = 1;
mapOut = mapInternal;
end

== matlab function QCar2_DetailedScenario-2025a/basicQCarIO/pointCloud/findXYContour ==
  data: distances input; X output size=720; heading input; Y output size=720; d_max input
function [X, Y] = findXYContour(distances, heading, d_max)

% find indices where distances corresponds to the d_max (bordering circle)
idx = distances < d_max;

% drop the bordering circle
temp_distances = distances(idx);
temp_heading = heading(idx);
% find X, Y pairs from distance, heading
X = temp_distances.*cos(temp_heading);
X_size = size(X);
Y = temp_distances.*sin(temp_heading);
Y_size = size(Y);

== matlab function QCar2_DetailedScenario-2025a/basicQCarIO/LidarScanMatchICP ==
  data: lidar_pts input; pose output; dt input; isNew output
function [pose, isNew] = LidarScanMatchICP(lidar_pts, dt)
% Simulation-only LiDAR odometry using scan-to-scan ICP.
% pose = [x; y; yaw]

%#codegen
coder.extrinsic('icp_tform_4x4');

% --- Persistent numeric memory (NO empties)
persistent prevPts3 hasPrev T_global
if isempty(hasPrev)
    hasPrev  = false;
    prevPts3 = zeros(360,3);   % fixed-size
    T_global = eye(4);         % fixed-size
end

% --- Fixed-size outputs so Simulink can compile
pose = zeros(3,1);
isNew = false;

% Force expected shape (helps if Simulink treats as 1-D)
lidar_pts = reshape(lidar_pts, 360, 2);

% Build fixed 360x3 (z=0)
currPts3 = zeros(360,3);
currPts3(:,1:2) = lidar_pts;

% First scan initializes
if ~hasPrev
    prevPts3 = currPts3;
    hasPrev = true;
    isNew = true;
    return;
end

% Call extrinsic ICP helper: returns curr->prev
T = eye(4);  %#ok<NASGU>  % fixed-size for inference
T = icp_tform_4x4(currPts3, prevPts3);

% Integrate motion: prev->curr = inv(curr->prev)
T_inc = inv(T);
T_global = T_global * T_inc;

% Translation in rigid3d/affine3d matrix is in last row
x = T_global(4,1);
y = T_global(4,2);
yaw = atan2(T_global(2,1), T_global(1,1));

pose(:) = [x; y; yaw];
isNew = true;

% Update memory
prevPts3 = currPts3;
end

== matlab function QCar2_DetailedScenario-2025a/basicQCarIO/EKF_Fuse ==
  settings: updateMethod=DISCRETE
  data: dt input; pose_out output; v_meas input; r_meas input; lidar_new input; lidar_pose input; ok output
function [pose_out, ok] = EKF_Fuse(dt, v_meas, r_meas, lidar_new, lidar_pose)
% EKF State: x = [X; Y; psi; v]
%#codegen

% ---- Force scalars (handles 1-D "vector with 1 element" signals)
dt        = double(dt(1));
v_meas    = double(v_meas(1));
r_meas    = double(r_meas(1));
lidar_new = logical(lidar_new(1));

% lidar_pose should be 3x1
lidar_pose = reshape(double(lidar_pose), 3, 1);

persistent x P initialized
if isempty(initialized)
    x = zeros(4,1); % [x;y;psi;v]
    P = diag([2^2, 2^2, (pi/2)^2, 1^2]);
    initialized = true;
end

% ---- Tunables
% IMPORTANT: use element-wise / scalar math (no matrix power)
q_xy  = (0.20*dt) * (0.20*dt);   % (m)^2 per step
q_psi = (0.03*dt) * (0.03*dt);   % (rad)^2 per step
q_v   = (0.80*dt) * (0.80*dt);   % (m/s)^2 per step
Q = diag([q_xy, q_xy, q_psi, q_v]);

R_v = 0.25 * 0.25;

% Avoid deg2rad() to keep it simple for codegen
sig_psi = 3*pi/180;
R_l = diag([0.10*0.10, 0.10*0.10, sig_psi*sig_psi]);

% ---- Predict
psi = x(3);
v   = x(4);

x_pred = x;
x_pred(1) = x(1) + v * dt * cos(psi);
x_pred(2) = x(2) + v * dt * sin(psi);
x_pred(3) = wrapToPi(x(3) + r_meas * dt);
% x_pred(4) stays v, corrected by wheel measurement

F = eye(4);
F(1,3) = -v * dt * sin(psi);
F(1,4) =  dt * cos(psi);
F(2,3) =  v * dt * cos(psi);
F(2,4) =  dt * sin(psi);

P = F*P*F.' + Q;

% ---- Update with wheel speed: z = v_meas
H_v = [0 0 0 1];
innov_v = v_meas - x_pred(4);
S = H_v*P*H_v.' + R_v;          % scalar
K = (P*H_v.') / S;              % 4x1
x_pred = x_pred + K*innov_v;
P = (eye(4) - K*H_v) * P;

% ---- Update with LiDAR pose: z = [x;y;psi]
if lidar_new
    H_l = [1 0 0 0;
           0 1 0 0;
           0 0 1 0];
    zhat  = x_pred(1:3);
    innov = lidar_pose - zhat;
    innov(3) = wrapToPi(innov(3));

    S = H_l*P*H_l.' + R_l;       % 3x3
    K = (P*H_l.') / S;           % 4x3
    x_pred = x_pred + K*innov;
    x_pred(3) = wrapToPi(x_pred(3));
    P = (eye(4) - K*H_l) * P;
end

x = x_pred;

pose_out = x(1:3);
ok = true;
end

function a = wrapToPi(x)
a = mod(x+pi, 2*pi) - pi;
end

== matlab function QCar2_DetailedScenario-2025a/basicQCarIO/LidarPolarToCartesian ==
  data: dist input; pts output; ang input
function pts = LidarPolarToCartesian(dist, ang)
% Convert polar LiDAR scan to Cartesian point cloud (fixed size)
% dist, ang: 360x1 (or 1-D 360) -> output pts: 360x2

%#codegen

% Force column vectors (handles 1-D 360 too)
dist = dist(:);
ang  = ang(:);

N = numel(dist);      % should be 360

% Preallocate fixed-size output
pts = zeros(N,2);

% Compute all points (no size change)
pts(:,1) = dist .* cos(ang);
pts(:,2) = dist .* sin(ang);

% Invalidate bad ranges WITHOUT changing size
valid = (dist > 0.10) & (dist < 20.0) & isfinite(dist) & isfinite(ang);
pts(~valid,:) = NaN;     % (or 0) but NaN is easier to filter later
end
